simulink subsystem "Earth"  (R2022a)
settings: Solver=VariableStepAuto  StartTime=0.0  StopTime=10.0  RelTol=1e-3
undefined symbols (not defined in the file or in its folder): sig_es
libraries: matrix_library x2, simulink_extras x1
settings Model: Creator=emmamarsden  LastModifiedBy=emmamarsden

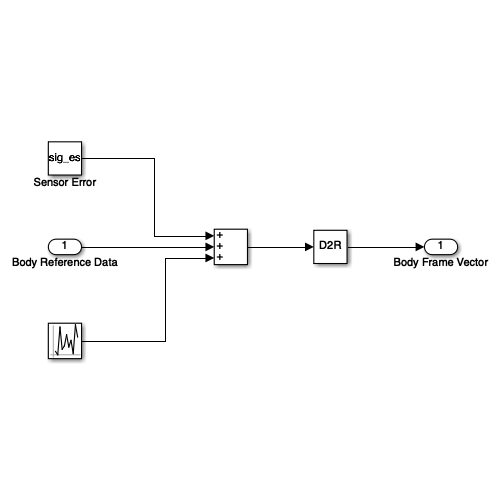
[thumbnail: Simulink's stored preview of the top-level diagram]
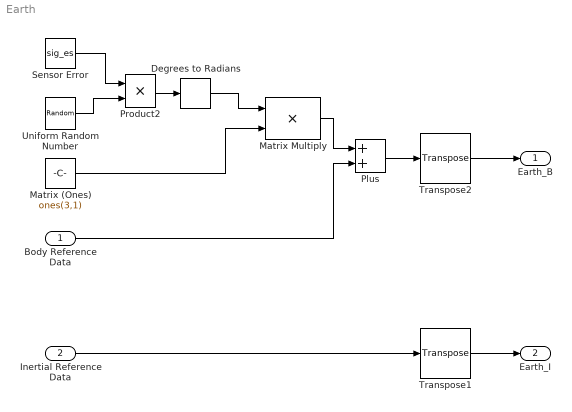
== system Earth ==
  Body Reference Data : Inport
  Inertial Reference Data : Inport  Port=2
  Degrees to Radians : simulink_extras/Transformations/Degrees to Radians
  Matrix (Ones) : Constant  Value=ones(3,1)  VectorParams1D=off
  Matrix Multiply : Product
  Plus : Sum
  Product2 : Product
  Sensor Error : Constant  Value=sig_es
  Transpose1 : matrix_library/Transpose
      settings: SourceProductBaseCode=SL
  Transpose2 : matrix_library/Transpose
      settings: SourceProductBaseCode=SL
  Uniform Random Number : UniformRandomNumber  SampleTime=0.1
  Earth_B : Outport
  Earth_I : Outport  Port=2
  wires:
  Inertial Reference Data/1 -> Transpose1/1
  Transpose1/1 -> Earth_I/1
  Sensor Error/1 -> Product2/1
  Uniform Random Number/1 -> Product2/2
  Matrix (Ones)/1 -> Matrix Multiply/2
  Matrix Multiply/1 -> Plus/1
  Degrees to Radians/1 -> Matrix Multiply/1
  Product2/1 -> Degrees to Radians/1
  Plus/1 -> Transpose2/1
  Transpose2/1 -> Earth_B/1
  Body Reference Data/1 -> Plus/2
